simulink model "Rocket_Code"  (R2020a)
settings: Solver=VariableStepAuto  StartTime=0.0  StopTime=10.0  RelTol=1e-3
undefined symbols (not defined in the file): KiPitchAttitude, KiPitchRate, KiRollAttitude, KiRollRate, KiYawRate, KpPitchAttitude, KpPitchRate, KpRollAttitude, KpRollRate, KpYawRate
libraries: simulink x6, aerolibobsolete x1, aerolibatmos2 x1, aerolibnav x1
settings Model: Creator=Shaan Heugly  LastModifiedBy=Shaan Heugly

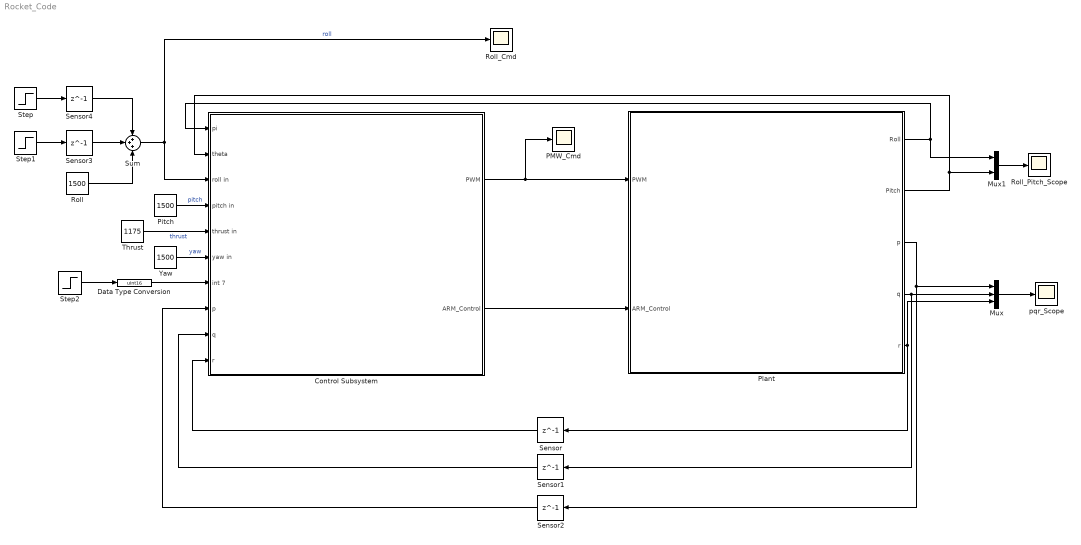
== system Rocket_Code ==
  Control Subsystem : Subsystem
  Data Type Conversion : DataTypeConversion  OutDataTypeStr=uint16
  Mux : Mux  Inputs=3
  Mux1 : Mux  Inputs=2
  PMW_Cmd : Scope
  Pitch : Constant  Value=1500  OutDataTypeStr=uint16
  Plant : Subsystem
  Roll : Constant  Value=1500
  Roll_Cmd : Scope
  Roll_Pitch_Scope : Scope
  Sensor{,1..4} (5 alike) : Delay  DelayLength=1
  Step : Step  Time=10  After=100  SampleTime=0
  Step1 : Step  Time=16  After=-100  SampleTime=0
  Step2 : Step  Time=5  Before=1499  After=1501  SampleTime=1/250
  Sum : Sum  Inputs=+++  OutDataTypeStr=uint16
  Thrust : Constant  Value=1175  OutDataTypeStr=uint16
  Yaw : Constant  Value=1500  OutDataTypeStr=uint16
  pqr_Scope : Scope
  wires:
  Control Subsystem/2(ARM_Control) -> Plant/2(ARM_Control)
  Control Subsystem/1(PWM) -> PMW_Cmd/1, Plant/1(PWM)
  Step/1 -> Sensor4/1
  Step1/1 -> Sensor3/1
  Sensor3/1 -> Sum/2
  Sensor4/1 -> Sum/1
  Roll/1 -> Sum/3
  Step2/1 -> Data Type Conversion/1
  Sum/1 -> Roll_Cmd/1, Control Subsystem/3(roll in)  "roll"
  Pitch/1 -> Control Subsystem/4(pitch in)  "pitch"
  Thrust/1 -> Control Subsystem/5(thrust in)  "thrust"
  Yaw/1 -> Control Subsystem/6(yaw in)  "yaw"
  Data Type Conversion/1 -> Control Subsystem/7(int 7)
  Plant/5(r) -> Mux/3, Sensor/1
  Sensor2/1 -> Control Subsystem/8(p)
  Sensor/1 -> Control Subsystem/10(r)
  Plant/4(q) -> Mux/2, Sensor1/1
  Sensor1/1 -> Control Subsystem/9(q)
  Plant/3(p) -> Sensor2/1, Mux/1
  Plant/2(Pitch) -> Control Subsystem/2(theta), Mux1/2
  Plant/1(Roll) -> Control Subsystem/1(pi), Mux1/1
  Mux1/1 -> Roll_Pitch_Scope/1
  Mux/1 -> pqr_Scope/1

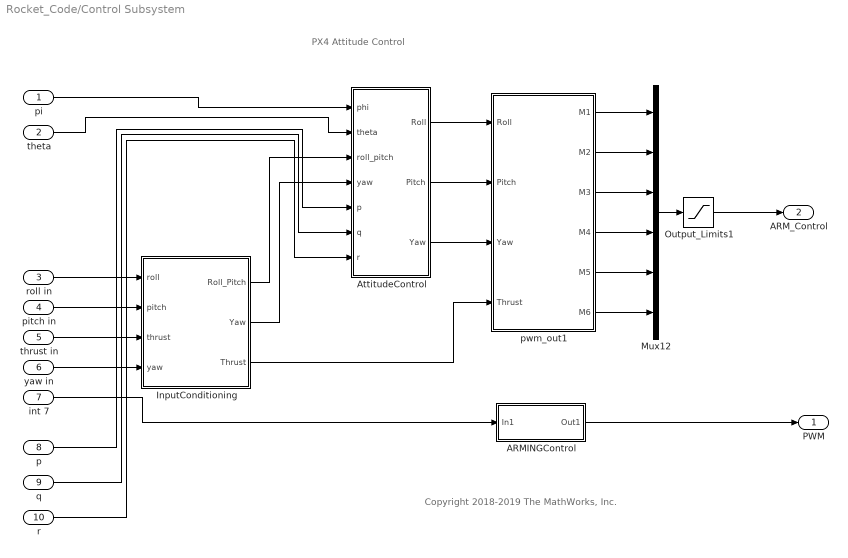
== system Rocket_Code/Control Subsystem ==
  note: Copyright 2018-2019 The MathWorks, Inc.
  note: PX4 Attitude Control
  pi : Inport
  theta : Inport  Port=2
  roll in : Inport  Port=3  OutDataTypeStr=uint16
  pitch in : Inport  Port=4  OutDataTypeStr=uint16
  thrust in : Inport  Port=5  OutDataTypeStr=uint16
  yaw in : Inport  Port=6  OutDataTypeStr=uint16
  int 7 : Inport  Port=7  OutDataTypeStr=uint16
  p : Inport  Port=8
  q : Inport  Port=9
  r : Inport  Port=10
  ARMINGControl : Subsystem
  AttitudeControl : Subsystem
  InputConditioning : Subsystem
  Mux12 : Mux  Inputs=6
  Output_Limits1 : Saturate  UpperLimit=2000  LowerLimit=1000
  pwm_out1 : MATLAB Function  TreatAsAtomicUnit=on  SystemSampleTime=0.004
  PWM : Outport  VectorParamsAs1DForOutWhenUnconnected=off
  ARM_Control : Outport  Port=2  VectorParamsAs1DForOutWhenUnconnected=off
  wires:
  r/1 -> AttitudeControl/7(r)
  InputConditioning/3(Thrust) -> pwm_out1/4(Thrust)
  pitch in/1 -> InputConditioning/2(pitch)
  int 7/1 -> ARMINGControl/1(In1)
  theta/1 -> AttitudeControl/2(theta)
  q/1 -> AttitudeControl/6(q)
  Output_Limits1/1 -> ARM_Control/1
  InputConditioning/1(Roll_Pitch) -> AttitudeControl/3(roll_pitch)
  pwm_out1/1(M1) -> Mux12/1
  pwm_out1/2(M2) -> Mux12/2
  p/1 -> AttitudeControl/5(p)
  AttitudeControl/3(Yaw) -> pwm_out1/3(Yaw)
  Mux12/1 -> Output_Limits1/1
  thrust in/1 -> InputConditioning/3(thrust)
  yaw in/1 -> InputConditioning/4(yaw)
  InputConditioning/2(Yaw) -> AttitudeControl/4(yaw)
  pwm_out1/3(M3) -> Mux12/3
  ARMINGControl/1(Out1) -> PWM/1
  AttitudeControl/1(Roll) -> pwm_out1/1(Roll)
  AttitudeControl/2(Pitch) -> pwm_out1/2(Pitch)
  pwm_out1/4(M4) -> Mux12/4
  pwm_out1/6(M6) -> Mux12/6
  roll in/1 -> InputConditioning/1(roll)
  pi/1 -> AttitudeControl/1(phi)
  pwm_out1/5(M5) -> Mux12/5

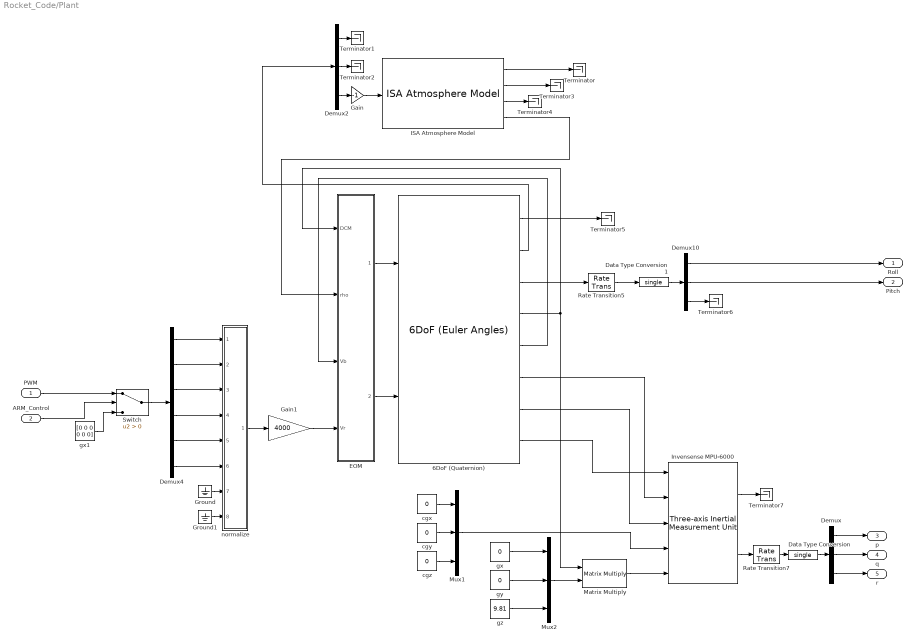
== system Rocket_Code/Plant ==
  PWM : Inport
  ARM_Control : Inport  Port=2
  6DoF (Quaternion) : aerolibobsolete/6DoF (Euler Angles)  units=Metric (MKS)  mtype=Fixed  rep=Quaternion  xme_0=[0 0 0]  Vm_0=[0 0 0]  eul_0=[0 0 0]  pm_0=[0 0 0]  mass_0=0.26  mass_e=0  mass_f=0  inertia=[0.00080, 0, 0; 0, 0.00065, 0; 0, 0, 0.0014]  inertia_e=eye(3)  inertia_f=eye(3)  k_quat=1.0
      settings: SourceProductBaseCode=AE
  Data Type Conversion : DataTypeConversion  OutDataTypeStr=single
  Data Type Conversion1 : DataTypeConversion  OutDataTypeStr=single
  Demux : Demux  Outputs=3
  Demux10 : Demux  Outputs=3
  Demux2 : Demux  Outputs=3
  Demux4 : Demux  Outputs=6
  EOM : Subsystem  mask{propD=0.1397, mass=0.26, vehiD=0.25, Cd=0.1}
      mask prompts: propD "Propeller Diameter"; mass "Vehicle Mass"; vehiD "Vehicle Diameter"; Cd "Drag Coefficient"
  Gain : Gain  Gain=-1
  Gain1 : Gain  Gain=4000
  Ground : Ground
  Ground1 : Ground
  ISA Atmosphere Model : aerolibatmos2/ISA Atmosphere Model  custom=on  g=9.80665  gamma=1.4  R=287.0531  L=0.0065  h_trop=11000  h_strat=20000  rho0=1.225  P0=101325  T0=288.15  h0=-10
  Invensense MPU-6000 : aerolibnav/Three-axis Inertial Measurement Unit  units=Metric (MKS)  imu=[0 0 0]  i_Ts=0.004  dtype_a=off  w_a=190  z_a=0.707  a_sf_cc=[0.98 0 0; 0 0.98 0; 0 0 0.98]  a_bias=[0 0 0]  a_sat="[-19.62  -19.62  -19.62 19.62 19.62 19.62]"  dtype_g=off  w_g=190  z_g=0.707  g_sf_cc=[.98 0 0; 0 .98 0; 0 0 .98]  g_bias=[0 0 0]  g_sens=[0 0 0]  g_sat="[-4.36  -4.36  -4.36 4.36 4.36 4.36]"  i_rand=on  i_seeds=[348631 366719 978432 189621 128794 214632]  i_pow=[0.0000001 0.0000001 0.0000001 0.0000000005 0.0000000005 0.0000000005]
  Matrix Multiply : Product  Multiplication=Matrix(*)
  Mux1 : Mux  Inputs=3
  Mux2 : Mux  Inputs=3
  Rate Transition5 : RateTransition  OutPortSampleTime=0.004
  Rate Transition7 : RateTransition  OutPortSampleTime=0.004
  Switch : Switch  Criteria=u2 > Threshold
  Terminator{,1..7} (8 alike) : Terminator
  cgx : Constant  Value=0
  cgy : Constant  Value=0
  cgz : Constant  Value=0
  gx : Constant  Value=0
  gx1 : Constant  Value=[0 0 0 0 0 0]  OutDataTypeStr=uint16
  gy : Constant  Value=0
  gz : Constant  Value=9.81
  normalize : Subsystem
      mask Display:
      | port_label('input', 1, 'pwm1');
      | port_label('input', 2, 'pwm2');
      | port_label('input', 3, 'pwm3');
      | port_label('input', 4, 'pwm4');
      | port_label('input', 5, 'pwm5');
      | port_label('input', 6, 'pwm6');
      | port_label('input', 7, 'pwm7');
      | port_label('input', 8, 'pwm8');
  Roll : Outport  VectorParamsAs1DForOutWhenUnconnected=off
  Pitch : Outport  Port=2  VectorParamsAs1DForOutWhenUnconnected=off
  p : Outport  Port=3  VectorParamsAs1DForOutWhenUnconnected=off
  q : Outport  Port=4  VectorParamsAs1DForOutWhenUnconnected=off
  r : Outport  Port=5  VectorParamsAs1DForOutWhenUnconnected=off
  wires:
  ISA Atmosphere Model/1 -> Terminator/1
  Demux10/1 -> Roll/1
  Rate Transition5/1 -> Data Type Conversion1/1
  Demux4/3 -> normalize/3(pwm3)
  6DoF (Quaternion)/8 -> Invensense MPU-6000/1
  PWM/1 -> Switch/1
  6DoF (Quaternion)/6 -> Invensense MPU-6000/2
  Rate Transition7/1 -> Data Type Conversion/1
  6DoF (Quaternion)/7 -> Invensense MPU-6000/3
  Mux2/1 -> Matrix Multiply/2
  ISA Atmosphere Model/3 -> Terminator4/1
  Ground1/1 -> normalize/8(pwm8)
  gx/1 -> Mux2/1
  Demux2/2 -> Terminator2/1
  Invensense MPU-6000/2 -> Rate Transition7/1
  Demux4/4 -> normalize/4(pwm4)
  6DoF (Quaternion)/3 -> Rate Transition5/1
  ISA Atmosphere Model/2 -> Terminator3/1
  Demux/1 -> p/1
  Ground/1 -> normalize/7(pwm7)
  Demux4/5 -> normalize/5(pwm5)
  Demux/3 -> r/1
  Mux1/1 -> Invensense MPU-6000/4
  6DoF (Quaternion)/4 -> EOM/1(DCM), Matrix Multiply/1
  6DoF (Quaternion)/5 -> EOM/3(Vb)
  6DoF (Quaternion)/1 -> Terminator5/1
  Switch/1 -> Demux4/1
  Invensense MPU-6000/1 -> Terminator7/1
  Data Type Conversion/1 -> Demux/1
  gx1/1 -> Switch/3
  Demux4/6 -> normalize/6(pwm6)
  Demux2/3 -> Gain/1
  Demux10/2 -> Pitch/1
  EOM/1(Forces) -> 6DoF (Quaternion)/1
  Demux4/1 -> normalize/1(pwm1)
  Data Type Conversion1/1 -> Demux10/1
  cgx/1 -> Mux1/1
  6DoF (Quaternion)/2 -> Demux2/1
  cgy/1 -> Mux1/2
  ISA Atmosphere Model/4 -> EOM/2(rho)
  Matrix Multiply/1 -> Invensense MPU-6000/5
  normalize/1(normalized_signals) -> Gain1/1
  cgz/1 -> Mux1/3
  EOM/2(moments) -> 6DoF (Quaternion)/2
  Demux4/2 -> normalize/2(pwm2)
  Gain/1 -> ISA Atmosphere Model/1
  gy/1 -> Mux2/2
  Demux2/1 -> Terminator1/1
  gz/1 -> Mux2/3
  ARM_Control/1 -> Switch/2
  Demux10/3 -> Terminator6/1
  Gain1/1 -> EOM/4(Vr)
  Demux/2 -> q/1

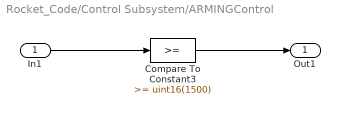
== system Rocket_Code/Control Subsystem/ARMINGControl ==
  In1 : Inport
  Compare To Constant3 : simulink/Logic and Bit Operations/Compare To Constant  relop=>=  const=uint16(1500)  OutDataTypeStr=boolean
  Out1 : Outport  VectorParamsAs1DForOutWhenUnconnected=off
  wires:
  Compare To Constant3/1 -> Out1/1
  In1/1 -> Compare To Constant3/1

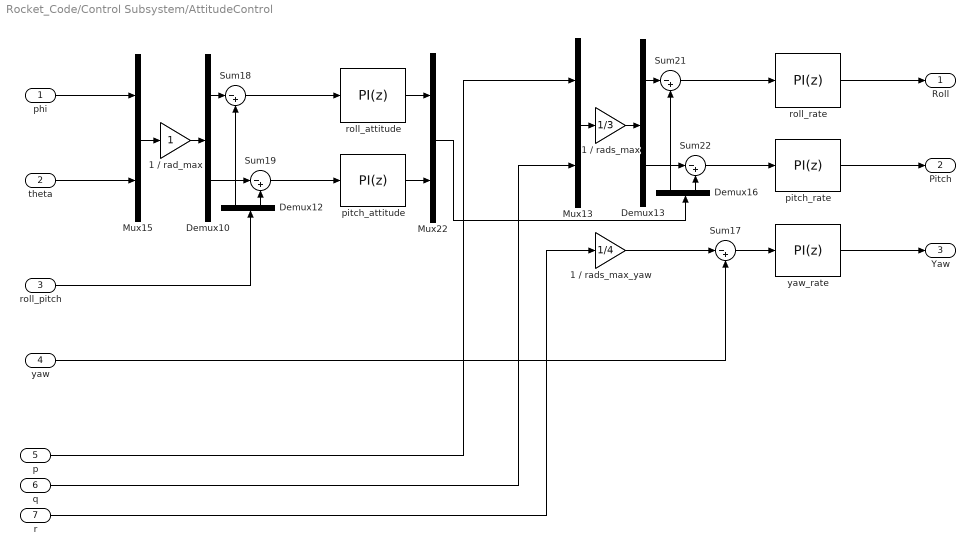
== system Rocket_Code/Control Subsystem/AttitudeControl ==
  phi : Inport
  theta : Inport  Port=2
  roll_pitch : Inport  Port=3
  yaw : Inport  Port=4
  p : Inport  Port=5
  q : Inport  Port=6
  r : Inport  Port=7
  1 / rad_max : Gain
  1 / rads_max : Gain  Gain=1/3
  1 / rads_max_yaw : Gain  Gain=1/4
  Demux{10,12..13,16} (4 alike) : Demux  Outputs=2
  Mux13 : Mux  Inputs=2
  Mux15 : Mux  Inputs=2
  Mux22 : Mux  Inputs=2
  Sum{17..19,21..22} (5 alike) : Sum  Inputs=|-+
  pitch_attitude : simulink/Continuous/PID Controller  Controller=PI  Form=Parallel  TimeDomain=Discrete-time  UseExternalTs=off  SampleTime=-1  IntegratorMethod=Forward Euler  FilterMethod=Forward Euler  ControllerParametersSource=internal  P=KpPitchAttitude  I=KiPitchAttitude  D=0.01  UseFilter=on  N=100  TunerSelectOption=Transfer Function Based (PID Tuner App)  InitialConditionSource=internal  InitialConditionForIntegrator=0  InitialConditionForFilter=0  DifferentiatorICPrevScaledInput=0  ExternalReset=none  TrackingMode=off  Kt=1  LimitOutput=on  UpperSaturationLimit=1  LowerSaturationLimit=-1  LinearizeAsGain=on  AntiWindupMode=back-calculation  Kb=1  POutMin=[]  POutMax=[]  IOutMin=[]  IOutMax=[]  DOutMin=[]  DOutMax=[]  NOutMin=[]  NOutMax=[]  SumOutMin=[]  SumOutMax=[]  SaturationOutMin=[]  SaturationOutMax=[]  PParamMin=[]  PParamMax=[]  IParamMin=[]  IParamMax=[]  DParamMin=[]  DParamMax=[]  NParamMin=[]  NParamMax=[]  KbParamMin=[]  KbParamMax=[]  KtParamMin=[]  KtParamMax=[]  KbOutMin=[]  KbOutMax=[]  KtOutMin=[]  KtOutMax=[]  IntegratorOutMin=[]  IntegratorOutMax=[]  FilterOutMin=[]  FilterOutMax=[]  SumI1OutMin=[]  SumI1OutMax=[]  SumI2OutMin=[]  SumI2OutMax=[]  SumI3OutMin=[]  SumI3OutMax=[]  SumI4OutMin=[]  SumI4OutMax=[]  SumDOutMin=[]  SumDOutMax=[]  DifferentiatorOutMin=[]  DifferentiatorOutMax=[]  FilterDiffOutCoefMin=[]  FilterDiffOutCoefMax=[]  ReciprocalOutMin=[]  ReciprocalOutMax=[]  SumDenOutMin=[]  SumDenOutMax=[]  SumNumOutMin=[]  SumNumOutMax=[]  DivideOutMin=[]  DivideOutMax=[]  UdiffTsProdOutMin=[]  UdiffTsProdOutMax=[]  NTsProdOutMin=[]  NTsProdOutMax=[]  UintegralTsProdOutMin=[]  UintegralTsProdOutMax=[]  UngainTsProdOutMin=[]  UngainTsProdOutMax=[]  IntegratorContinuousStateAttributes=''  IntegratorStateMustResolveToSignalObject=off  IntegratorRTWStateStorageClass=Auto  FilterContinuousStateAttributes=''  FilterStateMustResolveToSignalObject=off  FilterRTWStateStorageClass=Auto  ParallelPVariant=InternalParameters  IdealPVariant=Disabled  IVariant=InternalParameters  DVariant=Disabled  IntegratorVariant=Discrete  SatVariant=Enabled  AWVariant=BackCalculation  PCopyVariant=Disabled  TRVariant=Disabled  FdbkBlocksVariant=Forward  IdealPFdbkVariant=Disabled  SatFdbkVariant=Disabled  DerivativeFilterVariant=Disabled  NVariant=Disabled  NCopyVariant=Disabled_SignalSpec  FilterICVariant=Disabled  IntegratorICVariant=InternalICs  ExternalResetVariant=Disabled  TRSumVariant=Passthrough  SumFdbkVariant=Disabled  SumVariant=Sum_PI  TsampFilterVariant=InternalTs  TsampNgainVariant=Passthrough  TsampIntegralVariant=Passthrough
  pitch_rate : simulink/Continuous/PID Controller  Controller=PI  Form=Parallel  TimeDomain=Discrete-time  UseExternalTs=off  SampleTime=-1  IntegratorMethod=Forward Euler  FilterMethod=Forward Euler  ControllerParametersSource=internal  P=KpPitchRate  I=KiPitchRate  D=0.0024  UseFilter=on  N=100  TunerSelectOption=Transfer Function Based (PID Tuner App)  InitialConditionSource=internal  InitialConditionForIntegrator=0  InitialConditionForFilter=0  DifferentiatorICPrevScaledInput=0  ExternalReset=none  TrackingMode=off  Kt=1  LimitOutput=on  UpperSaturationLimit=1  LowerSaturationLimit=-1  LinearizeAsGain=on  AntiWindupMode=back-calculation  Kb=1  POutMin=[]  POutMax=[]  IOutMin=[]  IOutMax=[]  DOutMin=[]  DOutMax=[]  NOutMin=[]  NOutMax=[]  SumOutMin=[]  SumOutMax=[]  SaturationOutMin=[]  SaturationOutMax=[]  PParamMin=[]  PParamMax=[]  IParamMin=[]  IParamMax=[]  DParamMin=[]  DParamMax=[]  NParamMin=[]  NParamMax=[]  KbParamMin=[]  KbParamMax=[]  KtParamMin=[]  KtParamMax=[]  KbOutMin=[]  KbOutMax=[]  KtOutMin=[]  KtOutMax=[]  IntegratorOutMin=[]  IntegratorOutMax=[]  FilterOutMin=[]  FilterOutMax=[]  SumI1OutMin=[]  SumI1OutMax=[]  SumI2OutMin=[]  SumI2OutMax=[]  SumI3OutMin=[]  SumI3OutMax=[]  SumI4OutMin=[]  SumI4OutMax=[]  SumDOutMin=[]  SumDOutMax=[]  DifferentiatorOutMin=[]  DifferentiatorOutMax=[]  FilterDiffOutCoefMin=[]  FilterDiffOutCoefMax=[]  ReciprocalOutMin=[]  ReciprocalOutMax=[]  SumDenOutMin=[]  SumDenOutMax=[]  SumNumOutMin=[]  SumNumOutMax=[]  DivideOutMin=[]  DivideOutMax=[]  UdiffTsProdOutMin=[]  UdiffTsProdOutMax=[]  NTsProdOutMin=[]  NTsProdOutMax=[]  UintegralTsProdOutMin=[]  UintegralTsProdOutMax=[]  UngainTsProdOutMin=[]  UngainTsProdOutMax=[]  IntegratorContinuousStateAttributes=''  IntegratorStateMustResolveToSignalObject=off  IntegratorRTWStateStorageClass=Auto  FilterContinuousStateAttributes=''  FilterStateMustResolveToSignalObject=off  FilterRTWStateStorageClass=Auto  ParallelPVariant=InternalParameters  IdealPVariant=Disabled  IVariant=InternalParameters  DVariant=Disabled  IntegratorVariant=Discrete  SatVariant=Enabled  AWVariant=BackCalculation  PCopyVariant=Disabled  TRVariant=Disabled  FdbkBlocksVariant=Forward  IdealPFdbkVariant=Disabled  SatFdbkVariant=Disabled  DerivativeFilterVariant=Disabled  NVariant=Disabled  NCopyVariant=Disabled_SignalSpec  FilterICVariant=Disabled  IntegratorICVariant=InternalICs  ExternalResetVariant=Disabled  TRSumVariant=Passthrough  SumFdbkVariant=Disabled  SumVariant=Sum_PI  TsampFilterVariant=InternalTs  TsampNgainVariant=Passthrough  TsampIntegralVariant=Passthrough
  roll_attitude : simulink/Continuous/PID Controller  Controller=PI  Form=Parallel  TimeDomain=Discrete-time  UseExternalTs=off  SampleTime=-1  IntegratorMethod=Forward Euler  FilterMethod=Forward Euler  ControllerParametersSource=internal  P=KpRollAttitude  I=KiRollAttitude  D=0.01  UseFilter=on  N=100  TunerSelectOption=Transfer Function Based (PID Tuner App)  InitialConditionSource=internal  InitialConditionForIntegrator=0  InitialConditionForFilter=0  DifferentiatorICPrevScaledInput=0  ExternalReset=none  TrackingMode=off  Kt=1  LimitOutput=on  UpperSaturationLimit=1  LowerSaturationLimit=-1  LinearizeAsGain=on  AntiWindupMode=back-calculation  Kb=1  POutMin=[]  POutMax=[]  IOutMin=[]  IOutMax=[]  DOutMin=[]  DOutMax=[]  NOutMin=[]  NOutMax=[]  SumOutMin=[]  SumOutMax=[]  SaturationOutMin=[]  SaturationOutMax=[]  PParamMin=[]  PParamMax=[]  IParamMin=[]  IParamMax=[]  DParamMin=[]  DParamMax=[]  NParamMin=[]  NParamMax=[]  KbParamMin=[]  KbParamMax=[]  KtParamMin=[]  KtParamMax=[]  KbOutMin=[]  KbOutMax=[]  KtOutMin=[]  KtOutMax=[]  IntegratorOutMin=[]  IntegratorOutMax=[]  FilterOutMin=[]  FilterOutMax=[]  SumI1OutMin=[]  SumI1OutMax=[]  SumI2OutMin=[]  SumI2OutMax=[]  SumI3OutMin=[]  SumI3OutMax=[]  SumI4OutMin=[]  SumI4OutMax=[]  SumDOutMin=[]  SumDOutMax=[]  DifferentiatorOutMin=[]  DifferentiatorOutMax=[]  FilterDiffOutCoefMin=[]  FilterDiffOutCoefMax=[]  ReciprocalOutMin=[]  ReciprocalOutMax=[]  SumDenOutMin=[]  SumDenOutMax=[]  SumNumOutMin=[]  SumNumOutMax=[]  DivideOutMin=[]  DivideOutMax=[]  UdiffTsProdOutMin=[]  UdiffTsProdOutMax=[]  NTsProdOutMin=[]  NTsProdOutMax=[]  UintegralTsProdOutMin=[]  UintegralTsProdOutMax=[]  UngainTsProdOutMin=[]  UngainTsProdOutMax=[]  IntegratorContinuousStateAttributes=''  IntegratorStateMustResolveToSignalObject=off  IntegratorRTWStateStorageClass=Auto  FilterContinuousStateAttributes=''  FilterStateMustResolveToSignalObject=off  FilterRTWStateStorageClass=Auto  ParallelPVariant=InternalParameters  IdealPVariant=Disabled  IVariant=InternalParameters  DVariant=Disabled  IntegratorVariant=Discrete  SatVariant=Enabled  AWVariant=BackCalculation  PCopyVariant=Disabled  TRVariant=Disabled  FdbkBlocksVariant=Forward  IdealPFdbkVariant=Disabled  SatFdbkVariant=Disabled  DerivativeFilterVariant=Disabled  NVariant=Disabled  NCopyVariant=Disabled_SignalSpec  FilterICVariant=Disabled  IntegratorICVariant=InternalICs  ExternalResetVariant=Disabled  TRSumVariant=Passthrough  SumFdbkVariant=Disabled  SumVariant=Sum_PI  TsampFilterVariant=InternalTs  TsampNgainVariant=Passthrough  TsampIntegralVariant=Passthrough
  roll_rate : simulink/Continuous/PID Controller  Controller=PI  Form=Parallel  TimeDomain=Discrete-time  UseExternalTs=off  SampleTime=-1  IntegratorMethod=Forward Euler  FilterMethod=Forward Euler  ControllerParametersSource=internal  P=KpRollRate  I=KiRollRate  D=0.0024  UseFilter=on  N=100  TunerSelectOption=Transfer Function Based (PID Tuner App)  InitialConditionSource=internal  InitialConditionForIntegrator=0  InitialConditionForFilter=0  DifferentiatorICPrevScaledInput=0  ExternalReset=none  TrackingMode=off  Kt=1  LimitOutput=on  UpperSaturationLimit=1  LowerSaturationLimit=-1  LinearizeAsGain=on  AntiWindupMode=back-calculation  Kb=1  POutMin=[]  POutMax=[]  IOutMin=[]  IOutMax=[]  DOutMin=[]  DOutMax=[]  NOutMin=[]  NOutMax=[]  SumOutMin=[]  SumOutMax=[]  SaturationOutMin=[]  SaturationOutMax=[]  PParamMin=[]  PParamMax=[]  IParamMin=[]  IParamMax=[]  DParamMin=[]  DParamMax=[]  NParamMin=[]  NParamMax=[]  KbParamMin=[]  KbParamMax=[]  KtParamMin=[]  KtParamMax=[]  KbOutMin=[]  KbOutMax=[]  KtOutMin=[]  KtOutMax=[]  IntegratorOutMin=[]  IntegratorOutMax=[]  FilterOutMin=[]  FilterOutMax=[]  SumI1OutMin=[]  SumI1OutMax=[]  SumI2OutMin=[]  SumI2OutMax=[]  SumI3OutMin=[]  SumI3OutMax=[]  SumI4OutMin=[]  SumI4OutMax=[]  SumDOutMin=[]  SumDOutMax=[]  DifferentiatorOutMin=[]  DifferentiatorOutMax=[]  FilterDiffOutCoefMin=[]  FilterDiffOutCoefMax=[]  ReciprocalOutMin=[]  ReciprocalOutMax=[]  SumDenOutMin=[]  SumDenOutMax=[]  SumNumOutMin=[]  SumNumOutMax=[]  DivideOutMin=[]  DivideOutMax=[]  UdiffTsProdOutMin=[]  UdiffTsProdOutMax=[]  NTsProdOutMin=[]  NTsProdOutMax=[]  UintegralTsProdOutMin=[]  UintegralTsProdOutMax=[]  UngainTsProdOutMin=[]  UngainTsProdOutMax=[]  IntegratorContinuousStateAttributes=''  IntegratorStateMustResolveToSignalObject=off  IntegratorRTWStateStorageClass=Auto  FilterContinuousStateAttributes=''  FilterStateMustResolveToSignalObject=off  FilterRTWStateStorageClass=Auto  ParallelPVariant=InternalParameters  IdealPVariant=Disabled  IVariant=InternalParameters  DVariant=Disabled  IntegratorVariant=Discrete  SatVariant=Enabled  AWVariant=BackCalculation  PCopyVariant=Disabled  TRVariant=Disabled  FdbkBlocksVariant=Forward  IdealPFdbkVariant=Disabled  SatFdbkVariant=Disabled  DerivativeFilterVariant=Disabled  NVariant=Disabled  NCopyVariant=Disabled_SignalSpec  FilterICVariant=Disabled  IntegratorICVariant=InternalICs  ExternalResetVariant=Disabled  TRSumVariant=Passthrough  SumFdbkVariant=Disabled  SumVariant=Sum_PI  TsampFilterVariant=InternalTs  TsampNgainVariant=Passthrough  TsampIntegralVariant=Passthrough
  yaw_rate : simulink/Continuous/PID Controller  Controller=PI  Form=Parallel  TimeDomain=Discrete-time  UseExternalTs=off  SampleTime=-1  IntegratorMethod=Forward Euler  FilterMethod=Forward Euler  ControllerParametersSource=internal  P=KpYawRate  I=KiYawRate  D=0  UseFilter=on  N=100  TunerSelectOption=Transfer Function Based (PID Tuner App)  InitialConditionSource=internal  InitialConditionForIntegrator=0  InitialConditionForFilter=0  DifferentiatorICPrevScaledInput=0  ExternalReset=none  TrackingMode=off  Kt=1  LimitOutput=on  UpperSaturationLimit=1  LowerSaturationLimit=-1  LinearizeAsGain=on  AntiWindupMode=back-calculation  Kb=1  POutMin=[]  POutMax=[]  IOutMin=[]  IOutMax=[]  DOutMin=[]  DOutMax=[]  NOutMin=[]  NOutMax=[]  SumOutMin=[]  SumOutMax=[]  SaturationOutMin=[]  SaturationOutMax=[]  PParamMin=[]  PParamMax=[]  IParamMin=[]  IParamMax=[]  DParamMin=[]  DParamMax=[]  NParamMin=[]  NParamMax=[]  KbParamMin=[]  KbParamMax=[]  KtParamMin=[]  KtParamMax=[]  KbOutMin=[]  KbOutMax=[]  KtOutMin=[]  KtOutMax=[]  IntegratorOutMin=[]  IntegratorOutMax=[]  FilterOutMin=[]  FilterOutMax=[]  SumI1OutMin=[]  SumI1OutMax=[]  SumI2OutMin=[]  SumI2OutMax=[]  SumI3OutMin=[]  SumI3OutMax=[]  SumI4OutMin=[]  SumI4OutMax=[]  SumDOutMin=[]  SumDOutMax=[]  DifferentiatorOutMin=[]  DifferentiatorOutMax=[]  FilterDiffOutCoefMin=[]  FilterDiffOutCoefMax=[]  ReciprocalOutMin=[]  ReciprocalOutMax=[]  SumDenOutMin=[]  SumDenOutMax=[]  SumNumOutMin=[]  SumNumOutMax=[]  DivideOutMin=[]  DivideOutMax=[]  UdiffTsProdOutMin=[]  UdiffTsProdOutMax=[]  NTsProdOutMin=[]  NTsProdOutMax=[]  UintegralTsProdOutMin=[]  UintegralTsProdOutMax=[]  UngainTsProdOutMin=[]  UngainTsProdOutMax=[]  IntegratorContinuousStateAttributes=''  IntegratorStateMustResolveToSignalObject=off  IntegratorRTWStateStorageClass=Auto  FilterContinuousStateAttributes=''  FilterStateMustResolveToSignalObject=off  FilterRTWStateStorageClass=Auto  ParallelPVariant=InternalParameters  IdealPVariant=Disabled  IVariant=InternalParameters  DVariant=Disabled  IntegratorVariant=Discrete  SatVariant=Enabled  AWVariant=BackCalculation  PCopyVariant=Disabled  TRVariant=Disabled  FdbkBlocksVariant=Forward  IdealPFdbkVariant=Disabled  SatFdbkVariant=Disabled  DerivativeFilterVariant=Disabled  NVariant=Disabled  NCopyVariant=Disabled_SignalSpec  FilterICVariant=Disabled  IntegratorICVariant=InternalICs  ExternalResetVariant=Disabled  TRSumVariant=Passthrough  SumFdbkVariant=Disabled  SumVariant=Sum_PI  TsampFilterVariant=InternalTs  TsampNgainVariant=Passthrough  TsampIntegralVariant=Passthrough
  Roll : Outport  VectorParamsAs1DForOutWhenUnconnected=off
  Pitch : Outport  Port=2  VectorParamsAs1DForOutWhenUnconnected=off
  Yaw : Outport  Port=3  VectorParamsAs1DForOutWhenUnconnected=off
  wires:
  r/1 -> 1 / rads_max_yaw/1
  q/1 -> Mux13/2
  Mux22/1 -> Demux16/1
  yaw_rate/1 -> Yaw/1
  phi/1 -> Mux15/1
  Mux15/1 -> 1 / rad_max/1
  theta/1 -> Mux15/2
  1 / rads_max_yaw/1 -> Sum17/1
  roll_rate/1 -> Roll/1
  Sum19/1 -> pitch_attitude/1
  pitch_attitude/1 -> Mux22/2
  roll_attitude/1 -> Mux22/1
  Demux16/1 -> Sum21/2
  yaw/1 -> Sum17/2
  roll_pitch/1 -> Demux12/1
  Demux16/2 -> Sum22/2
  Demux12/1 -> Sum18/2
  Demux12/2 -> Sum19/2
  p/1 -> Mux13/1
  Demux10/1 -> Sum18/1
  Demux10/2 -> Sum19/1
  1 / rad_max/1 -> Demux10/1
  Sum18/1 -> roll_attitude/1
  pitch_rate/1 -> Pitch/1
  Mux13/1 -> 1 / rads_max/1
  Sum22/1 -> pitch_rate/1
  Sum17/1 -> yaw_rate/1
  Demux13/1 -> Sum21/1
  Demux13/2 -> Sum22/1
  1 / rads_max/1 -> Demux13/1
  Sum21/1 -> roll_rate/1

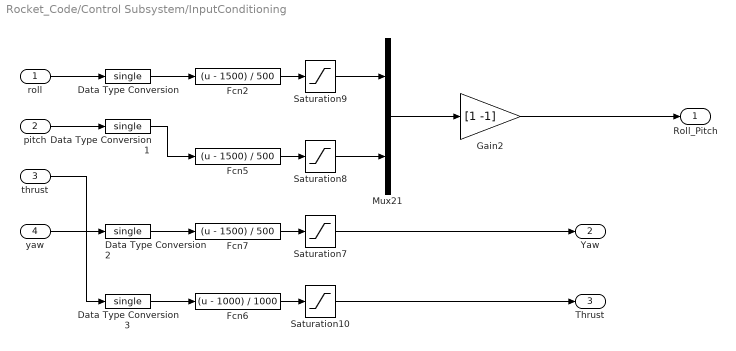
== system Rocket_Code/Control Subsystem/InputConditioning ==
  roll : Inport
  pitch : Inport  Port=2
  thrust : Inport  Port=3
  yaw : Inport  Port=4
  Data Type Conversion{,1..3} (4 alike) : DataTypeConversion  OutDataTypeStr=single
  Fcn2 : Fcn  Expr=(u - 1500) / 500
  Fcn5 : Fcn  Expr=(u - 1500) / 500
  Fcn6 : Fcn  Expr=(u - 1000) / 1000
  Fcn7 : Fcn  Expr=(u - 1500) / 500
  Gain2 : Gain  Gain=[1 -1]  OutDataTypeStr=Inherit: Inherit via back propagation
  Mux21 : Mux  Inputs=2
  Saturation10 : Saturate  UpperLimit=1  LowerLimit=0
  Saturation7 : Saturate  UpperLimit=1  LowerLimit=-1
  Saturation8 : Saturate  UpperLimit=1  LowerLimit=-1
  Saturation9 : Saturate  UpperLimit=1  LowerLimit=-1
  Roll_Pitch : Outport  VectorParamsAs1DForOutWhenUnconnected=off
  Yaw : Outport  Port=2  VectorParamsAs1DForOutWhenUnconnected=off
  Thrust : Outport  Port=3  VectorParamsAs1DForOutWhenUnconnected=off
  wires:
  Saturation10/1 -> Thrust/1
  Saturation7/1 -> Yaw/1
  Gain2/1 -> Roll_Pitch/1
  Mux21/1 -> Gain2/1
  Saturation8/1 -> Mux21/2
  Fcn6/1 -> Saturation10/1
  thrust/1 -> Data Type Conversion3/1
  Fcn2/1 -> Saturation9/1
  Fcn5/1 -> Saturation8/1
  Saturation9/1 -> Mux21/1
  Fcn7/1 -> Saturation7/1
  yaw/1 -> Data Type Conversion2/1
  pitch/1 -> Data Type Conversion1/1
  roll/1 -> Data Type Conversion/1
  Data Type Conversion/1 -> Fcn2/1
  Data Type Conversion1/1 -> Fcn5/1
  Data Type Conversion2/1 -> Fcn7/1
  Data Type Conversion3/1 -> Fcn6/1

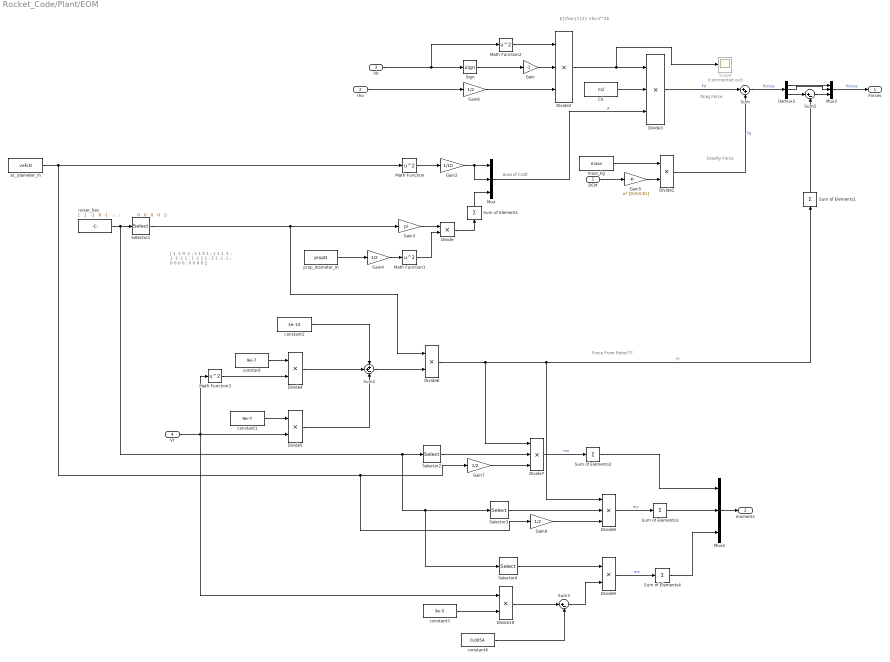
== system Rocket_Code/Plant/EOM ==
  note: Area of Craft
  note: [   1   -1    0   -1   ;
      |     1    1    0    1   ;
      |     1    1    1   -1   ;
      |     1   -1   -1    1   ;
      |     1   -1    1    1   ;
      |     1    1   -1   -1   ;
      |     0    0    0     0   ;
      |     0    0    0     0   ];
  note: Force From Rotor???
  note: Gravity Force
  note: Drag Force
  note: ${\frac{1}2} \rho V^2$
  DCM : Inport
  rho : Inport  Port=2
  Vb : Inport  Port=3
  Vr : Inport  Port=4
  Cd : Constant  Value=Cd
  Demux3 : Demux  Outputs=3
  Divide{,1,4..6,9..10} (7 alike) : Product  Inputs=**
  Divide{2..3,7..8} (4 alike) : Product  Inputs=***
  Gain : Gain  Gain=-1
  Gain2 : Gain  Gain=1/10
  Gain3 : Gain  Gain=pi
  Gain{4,6..8} (4 alike) : Gain  Gain=1/2
  Gain5 : Gain  Gain=[0;0;9.81]  Multiplication=Matrix(u*K)
  Math Function{,1..3} (4 alike) : Math  Operator=square  SignedPower=on  SaturateOnIntegerOverflow=on
  Mux : Mux  Inputs=3
  Mux3 : Mux  Inputs=3
  Mux4 : Mux  Inputs=3
  Scope : Scope  Commented=on
  Selector1 : Selector  NumberOfDimensions=2  InputPortWidth=[8 4]  IndexOptions=Index vector (dialog),Index vector (dialog)  Indices=[1:8],1  OutputSizes=1,1
  Selector2 : Selector  NumberOfDimensions=2  InputPortWidth=[8 4]  IndexOptions=Index vector (dialog),Index vector (dialog)  Indices=[1:8],2  OutputSizes=1,1
  Selector3 : Selector  NumberOfDimensions=2  InputPortWidth=[8 4]  IndexOptions=Index vector (dialog),Index vector (dialog)  Indices=[1:8],3  OutputSizes=1,1
  Selector4 : Selector  NumberOfDimensions=2  InputPortWidth=[8 4]  IndexOptions=Index vector (dialog),Index vector (dialog)  Indices=[1:8],4  OutputSizes=1,1
  Sign : Signum
  Sum : Sum  Inputs=|++
  Sum of Elements{,1..4} (5 alike) : Sum  Inputs=+
  Sum1 : Sum  Inputs=++-
  Sum2 : Sum  Inputs=|+-
  Sum3 : Sum  Inputs=|+-
  ac_diameter_m : Constant  Value=vehiD
  constant : Constant  Value=9e-7
  constant1 : Constant  Value=9e-7
  constant2 : Constant  Value=1e-14
  constant3 : Constant  Value=3e-5
  constant4 : Constant  Value=0.0054
  mass_kg : Constant  Value=mass
  mixer_hex : Constant  Value=|
      | [   1   -1   0  -1   ;
      |             1  1   0   1   ;
      |             1  1   1  -1   ;
      |             1  -1  -1   1   ;
      |             1   -1  1  1   ;
      |             1   1   -1   -1   ;
      |             0   0   0   0   ;
      |             0   0   0   0   ];
  prop_diameter_m : Constant  Value=propD
  Forces : Outport  VectorParamsAs1DForOutWhenUnconnected=off
  moments : Outport  Port=2  VectorParamsAs1DForOutWhenUnconnected=off
  wires:
  Math Function/1 -> Gain2/1
  Divide6/1 -> Divide7/1, Divide8/1, Sum of Elements1/1  "Fr"
  Sum/1 -> Demux3/1  "forces"
  constant/1 -> Divide4/1
  constant1/1 -> Divide5/1
  DCM/1 -> Gain5/1
  Divide3/1 -> Sum/1  "Fd"
  mass_kg/1 -> Divide1/1
  Gain5/1 -> Divide1/2
  Sum of Elements/1 -> Mux/3
  Cd/1 -> Divide3/2
  Math Function2/1 -> Divide2/1
  Gain4/1 -> Math Function1/1
  Gain3/1 -> Divide/1
  Divide1/1 -> Sum/2  "Fg"
  Selector1/1 -> Divide6/1, Gain3/1
  Divide/1 -> Sum of Elements/1
  Mux/1 -> Divide3/3  "A"
  prop_diameter_m/1 -> Gain4/1
  Gain6/1 -> Divide2/3
  Math Function1/1 -> Divide/2
  mixer_hex/1 -> Selector4/1, Selector3/1, Selector2/1, Selector1/1
  Gain2/1 -> Mux/2, Mux/1
  ac_diameter_m/1 -> Gain8/1, Gain7/1, Math Function/1
  Selector3/1 -> Divide8/2
  Sum2/1 -> Mux3/3
  Divide4/1 -> Sum1/2
  Vr/1 -> Divide10/1, Math Function3/1, Divide5/2
  Gain7/1 -> Divide7/3
  Sum1/1 -> Divide6/2
  Math Function3/1 -> Divide4/2
  constant2/1 -> Sum1/1
  Divide5/1 -> Sum1/3
  Sum of Elements3/1 -> Mux4/2
  Mux3/1 -> Forces/1  "forces"
  Selector2/1 -> Divide7/2
  Divide10/1 -> Sum3/1
  Demux3/3 -> Sum2/1
  constant4/1 -> Sum3/2
  Divide8/1 -> Sum of Elements3/1  "my"
  Demux3/1 -> Mux3/1
  Sum of Elements2/1 -> Mux4/1
  Selector4/1 -> Divide9/1
  Sum3/1 -> Divide9/2
  Demux3/2 -> Mux3/2
  Sum of Elements1/1 -> Sum2/2
  constant3/1 -> Divide10/2
  Divide7/1 -> Sum of Elements2/1  "mx"
  Gain8/1 -> Divide8/3
  Divide9/1 -> Sum of Elements4/1  "mz"
  Sum of Elements4/1 -> Mux4/3
  Mux4/1 -> moments/1
  Vb/1 -> Sign/1, Math Function2/1
  Divide2/1 -> Scope/1, Divide3/1
  rho/1 -> Gain6/1
  Gain/1 -> Divide2/2
  Sign/1 -> Gain/1

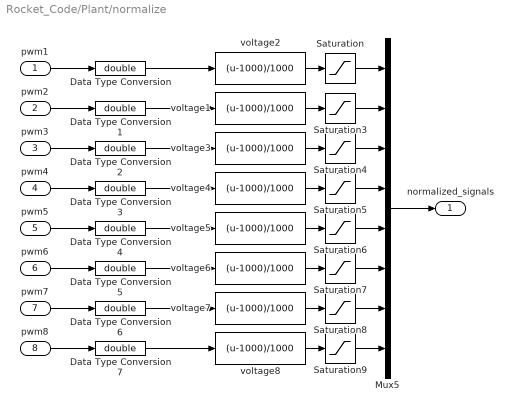
== system Rocket_Code/Plant/normalize ==
  pwm1 : Inport
  pwm2 : Inport  Port=2
  pwm3 : Inport  Port=3
  pwm4 : Inport  Port=4
  pwm5 : Inport  Port=5
  pwm6 : Inport  Port=6
  pwm7 : Inport  Port=7
  pwm8 : Inport  Port=8
  Data Type Conversion{,1..7} (8 alike) : DataTypeConversion  OutDataTypeStr=double
  Mux5 : Mux  Inputs=8
  Saturation{,3..9} (8 alike) : Saturate  UpperLimit=1  LowerLimit=0
  voltage{1..8} (8 alike) : Fcn  Expr=(u-1000)/1000
  normalized_signals : Outport  VectorParamsAs1DForOutWhenUnconnected=off
  wires:
  voltage1/1 -> Saturation3/1
  Saturation3/1 -> Mux5/2
  Saturation/1 -> Mux5/1
  Saturation6/1 -> Mux5/5
  voltage5/1 -> Saturation6/1
  pwm2/1 -> Data Type Conversion1/1
  pwm5/1 -> Data Type Conversion4/1
  pwm4/1 -> Data Type Conversion3/1
  pwm8/1 -> Data Type Conversion7/1
  pwm6/1 -> Data Type Conversion5/1
  pwm7/1 -> Data Type Conversion6/1
  Saturation4/1 -> Mux5/3
  voltage3/1 -> Saturation4/1
  pwm1/1 -> Data Type Conversion/1
  Mux5/1 -> normalized_signals/1
  pwm3/1 -> Data Type Conversion2/1
  Saturation9/1 -> Mux5/8
  voltage8/1 -> Saturation9/1
  Saturation8/1 -> Mux5/7
  voltage7/1 -> Saturation8/1
  voltage2/1 -> Saturation/1
  voltage4/1 -> Saturation5/1
  voltage6/1 -> Saturation7/1
  Saturation7/1 -> Mux5/6
  Saturation5/1 -> Mux5/4
  Data Type Conversion/1 -> voltage2/1
  Data Type Conversion1/1 -> voltage1/1
  Data Type Conversion2/1 -> voltage3/1
  Data Type Conversion3/1 -> voltage4/1
  Data Type Conversion4/1 -> voltage5/1
  Data Type Conversion5/1 -> voltage6/1
  Data Type Conversion6/1 -> voltage7/1
  Data Type Conversion7/1 -> voltage8/1

== matlab function Rocket_Code/Control Subsystem/pwm_out1 ==
  data: Roll input; M1 output; Pitch input; Yaw input; Thrust input; M2 output; M3 output; M4 output; M5 output; M6 output
function [M1, M2, M3, M4, M5, M6] = motor_mixer(Roll, Pitch, Yaw, Thrust)

idle_PWM = uint16(1000);

% Quad X
% M1 = ((Roll + Pitch - Yaw) / 2 * Thrust + Thrust) * 1000 + idle_PWM;
% M2 = ((-Roll + Pitch + Yaw) / 2 * Thrust + Thrust) * 1000 + idle_PWM;
% M3 = ((-Roll - Pitch - Yaw) / 2 * Thrust + Thrust) * 1000 + idle_PWM;
% M4 = ((Roll - Pitch + Yaw) / 2 * Thrust + Thrust) * 1000 + idle_PWM;
% M5 = 1000;
% M6 = 1000;
% M7 = 1000;
% M8 = 1000;

% Quad +
% M1 = ((Pitch - Yaw) * Thrust / 2 + Thrust) * 1000 + idle_PWM;
% M2 = ((-Roll + Yaw) * Thrust / 2 + Thrust) * 1000 + idle_PWM;
% M3 = ((-Pitch - Yaw) * Thrust / 2 + Thrust) * 1000 + idle_PWM;
% M4 = ((Roll + Yaw) * Thrust / 2 + Thrust) * 1000 + idle_PWM;
% M5 = 1000;
% M6 = 1000;
% M7 = 1000;
% M8 = 1000;

% Hex X
% M1 = ((Pitch + Roll / 2 - Yaw) * Thrust / 2 + Thrust) * 1000 + idle_PWM;
% M2 = ((Pitch - Roll / 2 + Yaw) * Thrust / 2 + Thrust) * 1000 + idle_PWM;
% M3 = ((-Roll - Yaw) * Thrust / 2 + Thrust) * 1000 + idle_PWM;
% M4 = ((-Pitch - Roll / 2 + Yaw) * Thrust / 2 + Thrust) * 1000 + idle_PWM;
% M5 = ((-Pitch + Roll / 2 - Yaw) * Thrust / 2 + Thrust) * 1000 + idle_PWM;
% M6 = ((Roll + Yaw) * Thrust / 2 + Thrust) * 1000 + idle_PWM;
% M7 = 1000;
% M8 = 1000;

% Hex X (From Adam)
M1 = uint16(single(((-Roll - Yaw) * Thrust / 3 + Thrust) * single(1000))) + idle_PWM;
M2 = uint16(single(((Roll + Yaw) * Thrust / 3 + Thrust) * single(1000))) + idle_PWM;
M3 = uint16(single(((Pitch + (Roll / 2) - Yaw) * Thrust / 3 + Thrust) * single(1000))) + idle_PWM;
M4 = uint16(single(((-Pitch - (Roll / 2) + Yaw) * Thrust / 3 + Thrust) * single(1000))) + idle_PWM;
M5 = uint16(single(((Pitch - (Roll / 2) + Yaw) * Thrust / 3 + Thrust) * single(1000))) + idle_PWM;
M6 = uint16(single(((-Pitch + (Roll / 2) - Yaw) * Thrust / 3 + Thrust) * single(1000))) + idle_PWM;

% Hex X (Version 2)
% Roll/Yaw
% M1 = ((-Roll - Yaw) * Thrust / 2 + Thrust) * 1000 + idle_PWM;
% M2 = ((Roll + Yaw) * Thrust / 2 + Thrust) * 1000 + idle_PWM;
% % + Pitch/Roll
% M6 = ((Pitch + Roll / 2 - Yaw) * Thrust / 2 + Thrust) * 1000 + idle_PWM;
% M4 = ((Pitch - Roll / 2 + Yaw) * Thrust / 2 + Thrust) * 1000 + idle_PWM;
% % - Pitch/Roll
% M5 = ((-Pitch - Roll / 2 + Yaw) * Thrust / 2 + Thrust) * 1000 + idle_PWM;
% M3 = ((-Pitch + Roll / 2 - Yaw) * Thrust / 2 + Thrust) * 1000 + idle_PWM;
